simulink model "untitled"  (R2017b)
settings: Solver=VariableStepAuto  StartTime=0.0  StopTime=10.0  RelTol=1e-3
values from neighbouring files (symbols this model uses):
  Te = T/M    (= 0.03125)    [Script.m]    (also in sixpistolets_script.m = 3.125e-06)
settings Model: Creator=aldebert  LastModifiedBy=aldebert

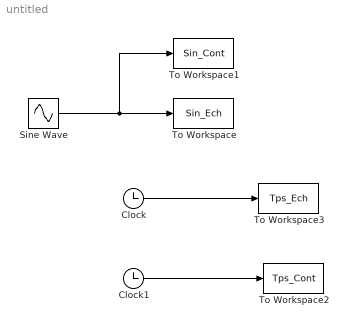
== system untitled ==
  Clock : Clock
  Clock1 : Clock
  Sine Wave : Sin  SampleTime=0
  To Workspace : ToWorkspace  VariableName=Sin_Ech  SampleTime=Te
  To Workspace1 : ToWorkspace  VariableName=Sin_Cont  SampleTime=Te/100
  To Workspace2 : ToWorkspace  VariableName=Tps_Cont  SampleTime=Te/100
  To Workspace3 : ToWorkspace  VariableName=Tps_Ech  SampleTime=Te
  wires:
  Sine Wave/1 -> To Workspace1/1, To Workspace/1
  Clock/1 -> To Workspace3/1
  Clock1/1 -> To Workspace2/1
